simulink model "PID0"  (R2015b)
settings: Solver=ode23t  StartTime=0.0  StopTime=2*360e-6  MaxStep=1e-7  MinStep=1e-9  RelTol=1e-3
values from neighbouring files (symbols this model uses):
  c2_val = I2_ripple/(8*f_sw*V2_ripple)    (= 3.125e-08)    [master_conv.m]
  delay_load = t1    (= 5.4e-06)    [master_conv.m]
  duty_inv = 100 - duty    (= 90)    [master_conv.m]
  duty_load = (t2-t1)/T_mach*100    (= 7)    [master_conv.m]
  Eg = 30    [master_conv.m]
  I_ref = 10    [master_conv.m]
  Kd1 = 0    [master_conv.m]
  Ki1 = 0    [master_conv.m]
  Kp1 = 10    [master_conv.m]
  l1_val = Vo1*(Vd_val-Vo1)/(I1_ripple*f_sw*Vd_val)    (= 5.09090909091e-05)    [master_conv.m]
  l2_val = V_ref*(Vd_val-V_ref)/(I2_ripple*f_sw*Vd_val)    (= 4.36363636364e-05)    [master_conv.m]
  r_val = 1    [master_conv.m]
  rc2_val = 0.0001    [master_conv.m]
  rl1_val = 0.0002    [master_conv.m]
  rl2_val = 0.0001    [master_conv.m]
  t2 = duty * T_mach / 100    (= 1.8e-05)    [master_conv.m]
  T_mach = 180e-6    (= 0.00018)    [master_conv.m]
  V_ref = 80    [master_conv.m]
  Vd_val = 110    [master_conv.m]
libraries: powerlib x33, powerlib_meascontrol x4, simulink x2
settings Model: Creator=Akshay  LastModifiedBy=Akshay
settings SolverCC: ZeroCrossAlgorithm=Adaptive
settings DataIOCC: SaveFormat=StructureWithTime
settings HardwareCC: ProdWordSize=32  ProdHWDeviceType=Specified

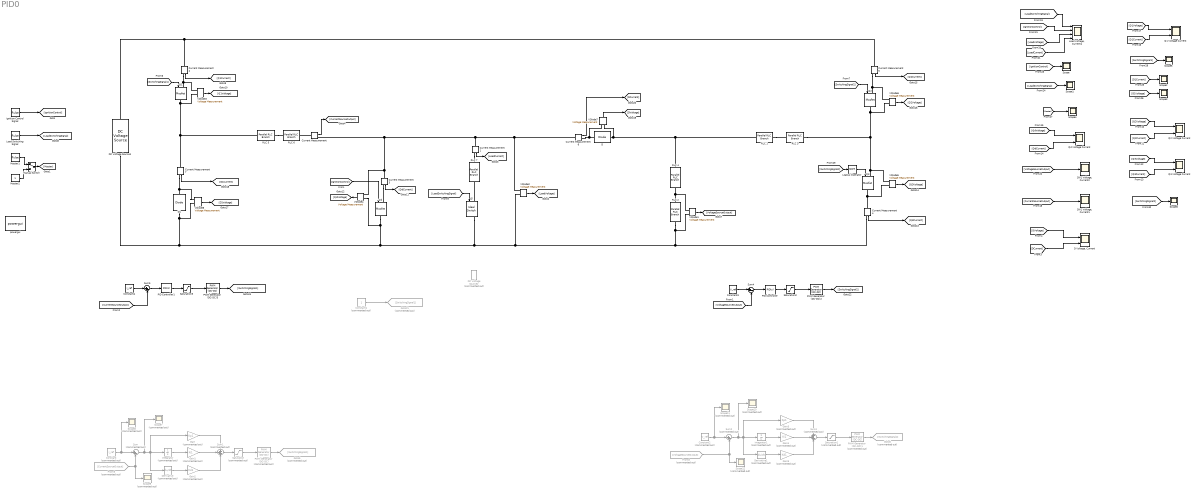
== system PID0 ==
  " RLC 1" : powerlib/Elements/Parallel RLC Branch  LConnTagsString=a  RConnTagsString=__new0  BranchType=R  Resistance=rl2_val  Inductance=5e-6  SetiL0=off  InitialCurrent=0  Capacitance=0.3e-6  Setx0=off  InitialVoltage=0  Measurements=None
  " RLC 2" : powerlib/Elements/Parallel RLC Branch  LConnTagsString=a  RConnTagsString=__new0  BranchType=C  Resistance=1  Inductance=1e-3  SetiL0=off  InitialCurrent=0  Capacitance=c2_val  Setx0=off  InitialVoltage=50  Measurements=None
  " RLC 3" : powerlib/Elements/Parallel RLC Branch  LConnTagsString=a  RConnTagsString=__new0  BranchType=L  Resistance=50  Inductance=l2_val  SetiL0=off  InitialCurrent=0  Capacitance=0.3e-6  Setx0=off  InitialVoltage=0  Measurements=None
  " RLC 4" : powerlib/Elements/Parallel RLC Branch  LConnTagsString=a  RConnTagsString=__new0  BranchType=R  Resistance=rc2_val  Inductance=1e-3  SetiL0=off  InitialCurrent=0  Capacitance=0.1e-6  Setx0=off  InitialVoltage=0  Measurements=None
  " RLC 5" : powerlib/Elements/Parallel RLC Branch  LConnTagsString=a  RConnTagsString=__new0  BranchType=R  Resistance=rl1_val  Inductance=5e-6  SetiL0=off  InitialCurrent=0  Capacitance=0.3e-6  Setx0=off  InitialVoltage=0  Measurements=None
  " RLC 6" : powerlib/Elements/Parallel RLC Branch  LConnTagsString=a  RConnTagsString=__new0  BranchType=L  Resistance=50  Inductance=l1_val  SetiL0=off  InitialCurrent=100  Capacitance=0.3e-6  Setx0=off  InitialVoltage=0  Measurements=None
  " RLC 7" : powerlib/Elements/Parallel RLC Branch  LConnTagsString=a  RConnTagsString=__new0  BranchType=R  Resistance=r_val  Inductance=1e-3  SetiL0=off  InitialCurrent=0  Capacitance=0.1e-6  Setx0=off  InitialVoltage=0  Measurements=None
  Constant : Constant  Commented=on  Value=I_ref
  Constant1 : Constant  Commented=on
  Constant2 : Constant  Commented=on  Value=V_ref
  Constant3 : Constant  Value=V_ref
  Constant4 : Constant  Value=I_ref
  Current Measurement{,1..7} (8 alike) : powerlib/Measurements/Current Measurement  PhasorSimulation=off  OutputType=Complex  PSBequivalent=0
  D : powerlib/Power Electronics/Diode  Ron=0.001  Lon=0  Vf=0.8  IC=0  UseSnubber=off  Rs=500  Cs=250e-9  Measurements=off
  "D Voltage, Current" : Scope  NumInputPorts=2
  D1 : powerlib/Power Electronics/Diode  Ron=0.001  Lon=0  Vf=0.8  IC=0  UseSnubber=off  Rs=500  Cs=250e-9  Measurements=off
  DC Voltage Source1 : powerlib/Electrical Sources/DC Voltage Source  Amplitude=Vd_val  Measurements=Voltage
  DC Voltage Source2 : powerlib/Electrical Sources/DC Voltage Source  Commented=on  Amplitude=Eg  Measurements=Voltage
  Derivative : Derivative  Commented=on
  Derivative1 : Derivative  Commented=on
  From5 : From  Commented=on  GotoTag=CurrentSourceOutput
  From8 : From  Commented=on  GotoTag=VoltageSourceOutput
  Gain : Gain  Commented=on  Gain=Kp1
  Gain1 : Gain  Commented=on  Gain=Ki1
  Gain2 : Gain  Commented=on  Gain=Kd1
  Gain3 : Gain  Commented=on  Gain=Kp1
  Gain4 : Gain  Commented=on  Gain=Ki1
  Gain5 : Gain  Commented=on  Gain=Kd1
  Goto21 : Goto  Commented=on  GotoTag=SwitchingSignal1
  Goto5 : Goto  Commented=on  GotoTag=SwitchingSignal1
  Goto6 : Goto  Commented=on  GotoTag=SwitchingSignal2
  Ignition Control Signal : DiscretePulseGenerator  PulseType=Time based  Period=T_mach  PulseWidth=duty_inv  PhaseDelay=t2-1.8e-6
  Integrator : Integrator  Commented=on
  Integrator1 : Integrator  Commented=on
  Load Switching Signal : DiscretePulseGenerator  PulseType=Time based  Period=T_mach  PulseWidth=duty_load  PhaseDelay=delay_load
  "Load Voltage, Current1" : Scope  NumInputPorts=4
  Logical Operator : Logic  Operator=NOT  AllPortsSameDT=off  OutDataTypeStr=boolean
  Manual Switch : ManualSwitch
  Master1 : DiscretePulseGenerator  PulseType=Time based  Period=180e-6  PulseWidth=6
  Master2 : Constant
  PID Controller : simulink/Continuous/PID Controller  Controller=PID  TimeDomain=Continuous-time  SampleTime=-1  IntegratorMethod=Forward Euler  FilterMethod=Forward Euler  Form=Parallel  UseFilter=on  ControllerParametersSource=internal  P=0.0123263661918898  I=446.876043850253  D=7.55447048769185e-08  N=710185400.04365  InitialConditionSource=internal  InitialConditionForIntegrator=0  InitialConditionForFilter=0  ExternalReset=none  LimitOutput=off  UpperSaturationLimit=inf  LowerSaturationLimit=-inf  LinearizeAsGain=on  AntiWindupMode=none  Kb=1  TrackingMode=off  Kt=1  PParamMin=[]  PParamMax=[]  IParamMin=[]  IParamMax=[]  DParamMin=[]  DParamMax=[]  NParamMin=[]  NParamMax=[]  KbParamMin=[]  KbParamMax=[]  KtParamMin=[]  KtParamMax=[]  POutMin=[]  POutMax=[]  IOutMin=[]  IOutMax=[]  DOutMin=[]  DOutMax=[]  NOutMin=[]  NOutMax=[]  KbOutMin=[]  KbOutMax=[]  KtOutMin=[]  KtOutMax=[]  IntegratorOutMin=[]  IntegratorOutMax=[]  FilterOutMin=[]  FilterOutMax=[]  SumOutMin=[]  SumOutMax=[]  SumI1OutMin=[]  SumI1OutMax=[]  SumI2OutMin=[]  SumI2OutMax=[]  SumI3OutMin=[]  SumI3OutMax=[]  SumDOutMin=[]  SumDOutMax=[]  SaturationOutMin=[]  SaturationOutMax=[]  IntegratorContinuousStateAttributes=''  IntegratorStateMustResolveToSignalObject=off  IntegratorRTWStateStorageClass=Auto  FilterContinuousStateAttributes=''  FilterStateMustResolveToSignalObject=off  FilterRTWStateStorageClass=Auto  DifferentiatorICPrevScaledInput=0  DifferentiatorOutMin=[]  DifferentiatorOutMax=[]
  PID Controller1 : simulink/Continuous/PID Controller  Controller=PID  TimeDomain=Continuous-time  SampleTime=-1  IntegratorMethod=Forward Euler  FilterMethod=Forward Euler  Form=Parallel  UseFilter=on  ControllerParametersSource=internal  P=0.0966437260550035  I=5969.79704533496  D=-9.61395268908695e-08  N=362743.333180625  InitialConditionSource=internal  InitialConditionForIntegrator=0  InitialConditionForFilter=0  ExternalReset=none  LimitOutput=off  UpperSaturationLimit=inf  LowerSaturationLimit=-inf  LinearizeAsGain=on  AntiWindupMode=none  Kb=1  TrackingMode=off  Kt=1  PParamMin=[]  PParamMax=[]  IParamMin=[]  IParamMax=[]  DParamMin=[]  DParamMax=[]  NParamMin=[]  NParamMax=[]  KbParamMin=[]  KbParamMax=[]  KtParamMin=[]  KtParamMax=[]  POutMin=[]  POutMax=[]  IOutMin=[]  IOutMax=[]  DOutMin=[]  DOutMax=[]  NOutMin=[]  NOutMax=[]  KbOutMin=[]  KbOutMax=[]  KtOutMin=[]  KtOutMax=[]  IntegratorOutMin=[]  IntegratorOutMax=[]  FilterOutMin=[]  FilterOutMax=[]  SumOutMin=[]  SumOutMax=[]  SumI1OutMin=[]  SumI1OutMax=[]  SumI2OutMin=[]  SumI2OutMax=[]  SumI3OutMin=[]  SumI3OutMax=[]  SumDOutMin=[]  SumDOutMax=[]  SaturationOutMin=[]  SaturationOutMax=[]  IntegratorContinuousStateAttributes=''  IntegratorStateMustResolveToSignalObject=off  IntegratorRTWStateStorageClass=Auto  FilterContinuousStateAttributes=''  FilterStateMustResolveToSignalObject=off  FilterRTWStateStorageClass=Auto  DifferentiatorICPrevScaledInput=0  DifferentiatorOutMin=[]  DifferentiatorOutMax=[]
  PWM Generator (DC-DC) : powerlib_meascontrol/Pulse & Signal Generators/PWM Generator (DC-DC)  Commented=on  Fsw=5000  Ts=0
  PWM Generator (DC-DC)1 : powerlib_meascontrol/Pulse & Signal Generators/PWM Generator (DC-DC)  Commented=on  Fsw=5000  Ts=0
  PWM Generator (DC-DC)2 : powerlib_meascontrol/Pulse & Signal Generators/PWM Generator (DC-DC)  Fsw=1000e3  Ts=0
  PWM Generator (DC-DC)3 : powerlib_meascontrol/Pulse & Signal Generators/PWM Generator (DC-DC)  Fsw=1000e3  Ts=0
  Q1 : powerlib/Power Electronics/Mosfet  Ron=0.00001  Lon=0  Rd=0.0000000000001  Vfd=0  IC=0  Rs=1e5  Cs=inf  Measurements=off
  Q1 Voltage Current : Scope  NumInputPorts=2
  Q2 : powerlib/Power Electronics/Mosfet  Ron=0.00001  Lon=0  Rd=0.0000000000001  Vfd=0  IC=0  Rs=1e5  Cs=inf  Measurements=off
  Q2 Voltage Current : Scope  NumInputPorts=2
  Q3 : powerlib/Power Electronics/Mosfet  Ron=0.00001  Lon=0  Rd=0.0000000000001  Vfd=0  IC=0  Rs=1e5  Cs=inf  Measurements=off
  Q3 Voltage Current : Scope  NumInputPorts=2
  Qd : powerlib/Power Electronics/Mosfet  Ron=0.00001  Lon=0  Rd=0.0000000000001  Vfd=0  IC=0  Rs=1e5  Cs=inf  Measurements=off
  Qd Voltage Current : Scope  NumInputPorts=2
  Ql : powerlib/Power Electronics/Ideal Switch  Ron=0.001  Lon=0  IC=0  Rs=1e5  Cs=inf  Measurements=on
  "SW1 Voltage, Current1" : Scope
  "SW1 Voltage, Current2" : Scope
  Saturation : Saturate  Commented=on  UpperLimit=0.99  LowerLimit=0
  Saturation1 : Saturate  Commented=on  UpperLimit=0.99  LowerLimit=0
  Saturation2 : Saturate  UpperLimit=0.99  LowerLimit=0
  Saturation3 : Saturate  UpperLimit=0.99  LowerLimit=0
  Scope{,1..6} (7 alike) : Scope
  Scope{7..12} (6 alike) : Scope  Commented=on
  Sum : Sum  Commented=on  Inputs=|+-
  Sum1 : Sum  Commented=on  Inputs=+++
  Sum2 : Sum  Commented=on  Inputs=|+-
  Sum3 : Sum  Commented=on  Inputs=+++
  Sum4 : Sum  Inputs=|+-
  Sum5 : Sum  Inputs=|+-
  VDiode{1..8} (8 alike) : powerlib/Measurements/Voltage Measurement  PhasorSimulation=off  OutputType=Complex  PSBequivalent=0
  powergui : powerlib/powergui  Priority=1  SimulationMode=Continuous  SolverType=Backward Euler  SampleTime=5e-07  frequency=60  SPID=on  DisableSnubberDevices=off  DisableRonSwitches=off  DisableVfSwitches=off  SwTol=0  DisplayEquations=off  Interpol=off  ExternalGateDelay=off  methode=off  Ts=0  FunctionMessages=off  echomessages=off  HookPort=off  EnableUseOfTLC=off  x0status=zero  frequencyindice=0  Pbase=100e6  ErrMax=1e-4  Iterations=50  UnitsV=kV  UnitsW=MW  buscounter=0  RestoreLinks=warning  ResistiveCurrentMeasurement=off  Frange=[0:2:500]  Ylog=off  Xlog=on  ShowGrid=off  save=off  variable=ZData  structure=ScopeData  ZoomFFT=off  StartTime=0.0  cycles=5  DisplayStyle=2  fundamental=50  FreqAxis=off  MaxFrequency=50000  frequencyindicesteady=1  RmsSteady=1  display=off
  wires:
  Logical Operator/1 -> Q3/1
  VDiode1/1 -> [VoltageSourceOutput]
  Ignition Control Signal/1 -> [IgnitionControl]
  [IgnitionControl] -> Qd/1
  VDiode2/1 -> [LoadVoltage]
  Current Measurement1/1 -> [LoadCurrent]
  Current Measurement/1 -> [CurrentSourceOutput]
  [SwitchingSignal1] -> Q1/1
  [SwitchingSignal2] -> Q2/1
  Load Switching Signal/1 -> [LoadSwitchingSignal]
  Manual Switch/1 -> [Master]
  Master1/1 -> Manual Switch/1
  Master2/1 -> Manual Switch/2
  Current Measurement2/1 -> [Q1Current]
  VDiode3/1 -> [Q1Voltage]
  Current Measurement3/1 -> [QdCurrent]
  VDiode4/1 -> [QdVoltage]
  Current Measurement4/1 -> [Q3Current]
  VDiode5/1 -> [Q3Voltage]
  VDiode6/1 -> [Q2Voltage]
  Current Measurement5/1 -> [Q2Current]
  [Q2Voltage] -> Q2 Voltage Current/1
  [Q2Current] -> Q2 Voltage Current/2
  [Q3Voltage] -> Q3 Voltage Current/1
  [Q3Current] -> Q3 Voltage Current/2
  [Q1Voltage] -> Q1 Voltage Current/1
  [Q1Current] -> Q1 Voltage Current/2
  [QdVoltage] -> Qd Voltage Current/1
  [QdCurrent] -> Qd Voltage Current/2
  [LoadSwitchingSignal] -> "Load Voltage, Current1"/1
  [VoltageSourceOutput] -> "SW1 Voltage, Current2"/1
  [IgnitionControl] -> Scope/1
  [LoadSwitchingSignal] -> Scope1/1
  [CurrentSourceOutput] -> "SW1 Voltage, Current1"/1
  Current Measurement7/1 -> [D1Current]
  VDiode8/1 -> [D1Voltage]
  [D1Current] -> Scope2/1
  [D1Voltage] -> Scope3/1
  [Master] -> Scope4/1
  [SwitchingSignal1] -> Scope5/1
  VDiode7/1 -> [DVoltage]
  Current Measurement6/1 -> [DCurrent]
  [DVoltage] -> "D Voltage, Current"/1
  [DCurrent] -> "D Voltage, Current"/2
  [SwitchingSignal2] -> Logical Operator/1
  [SwitchingSignal2] -> Scope6/1
  Constant/1 -> Scope8/1, Sum/1
  From5/1 -> Scope9/1, Sum/2
  Sum/1 -> Scope7/1, Derivative/1, Integrator/1, Gain/1
  Integrator/1 -> Gain1/1
  Derivative/1 -> Gain2/1
  Gain1/1 -> Sum1/2
  Gain/1 -> Sum1/1
  Gain2/1 -> Sum1/3
  Sum1/1 -> Saturation/1
  Saturation/1 -> PWM Generator (DC-DC)/1
  PWM Generator (DC-DC)/1 -> Goto5/1
  Constant1/1 -> Goto21/1
  Constant2/1 -> Scope11/1, Sum2/1
  From8/1 -> Sum2/2, Scope12/1
  Sum2/1 -> Scope10/1, Derivative1/1, Integrator1/1, Gain3/1
  Integrator1/1 -> Gain4/1
  Derivative1/1 -> Gain5/1
  Gain4/1 -> Sum3/2
  Gain3/1 -> Sum3/1
  Gain5/1 -> Sum3/3
  Sum3/1 -> Saturation1/1
  Saturation1/1 -> PWM Generator (DC-DC)1/1
  PWM Generator (DC-DC)1/1 -> Goto6/1
  Sum4/1 -> PID Controller/1
  Constant3/1 -> Sum4/1
  [VoltageSourceOutput] -> Sum4/2
  PID Controller/1 -> Saturation2/1
  Saturation2/1 -> PWM Generator (DC-DC)2/1
  PWM Generator (DC-DC)2/1 -> [SwitchingSignal2]
  Sum5/1 -> PID Controller1/1
  Constant4/1 -> Sum5/1
  [CurrentSourceOutput] -> Sum5/2
  PID Controller1/1 -> Saturation3/1
  Saturation3/1 -> PWM Generator (DC-DC)3/1
  PWM Generator (DC-DC)3/1 -> [SwitchingSignal1]
  [LoadSwitchingSignal] -> Ql/1
  [LoadVoltage] -> "Load Voltage, Current1"/3
  [LoadCurrent] -> "Load Voltage, Current1"/4
  [IgnitionControl] -> "Load Voltage, Current1"/2
  connections:
  " RLC 3"/RConn1 -- Q2/RConn1 -- VDiode6/LConn2 -- Q3/LConn1 -- VDiode5/LConn1
  " RLC 2"/LConn1 -- " RLC 4"/RConn1 -- VDiode1/LConn1
  VDiode7/LConn2 -- D/RConn1 -- " RLC 4"/LConn1 -- " RLC 1"/LConn1
  " RLC 1"/RConn1 -- " RLC 3"/LConn1
  VDiode3/LConn2 -- Q1/RConn1 -- Current Measurement7/LConn1 -- " RLC 5"/LConn1
  DC Voltage Source1/RConn1 -- Current Measurement5/LConn1 -- Current Measurement2/LConn1
  " RLC 5"/RConn1 -- " RLC 6"/LConn1
  Current Measurement/LConn1 -- " RLC 6"/RConn1
  Current Measurement3/LConn1 -- Current Measurement6/LConn1 -- VDiode2/LConn1 -- Current Measurement1/LConn1 -- Current Measurement/RConn1 -- VDiode4/LConn2
  Current Measurement2/RConn1 -- VDiode3/LConn1 -- Q1/LConn1
  Current Measurement3/RConn1 -- Qd/LConn1
  Current Measurement4/LConn1 -- Q3/RConn1 -- VDiode5/LConn2
  Current Measurement5/RConn1 -- VDiode6/LConn1 -- Q2/LConn1
  Current Measurement6/RConn1 -- D/LConn1 -- VDiode7/LConn1
  Current Measurement7/RConn1 -- D1/RConn1 -- VDiode8/LConn1
  Current Measurement1/RConn1 -- " RLC 7"/LConn1
  " RLC 2"/RConn1 -- VDiode1/LConn2 -- Ql/RConn1 -- VDiode8/LConn2 -- D1/LConn1 -- DC Voltage Source1/LConn1 -- VDiode4/LConn1 -- Qd/RConn1 -- VDiode2/LConn2 -- Current Measurement4/RConn1
  Ql/LConn1 -- " RLC 7"/RConn1
